simulink model "integrator_demo"  (Simulink 6.3)
settings: Solver=ode45  StartTime=0.0  StopTime=10.0  RelTol=1e-3
settings Model: LastModifiedBy=Ms1

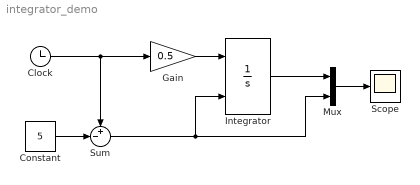
== system integrator_demo ==
  Clock : Clock
      settings: Decimation=10
  Constant : Constant  Value=5
  Gain : Gain  Gain=0.5  SaturateOnIntegerOverflow=on
  Integrator : Integrator  ExternalReset=rising  InitialCondition=10
  Mux : Mux  Inputs=2
  Scope : Scope
  Sum : Sum  Inputs=+-|  SaturateOnIntegerOverflow=on  InputSameDT=on
  wires:
  Mux/1 -> Scope/1
  Clock/1 -> Gain/1, Sum/1
  Integrator/1 -> Mux/1
  Sum/1 -> Mux/2, Integrator/2
  Gain/1 -> Integrator/1
  Constant/1 -> Sum/2
